simulink model "CompensadorDigitalCorrerArchivoM"  (R2018a)
settings: Solver=VariableStepAuto  StartTime=0.0  StopTime=10.0  RelTol=1e-3
undefined symbols (not defined in the file or in its folder): gcompensado, Gtotalw, integradorDigital
settings Model: Creator=Ignacio  LastModifiedBy=Ignacio

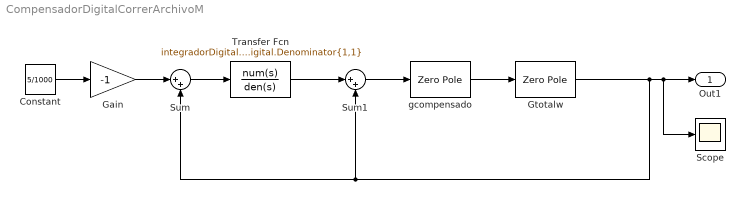
== system CompensadorDigitalCorrerArchivoM ==
  Constant : Constant  Value=5/1000
  Gain : Gain  Gain=-1
  Gtotalw : ZeroPole  Zeros=Gtotalw.Z{1,1}  Poles=Gtotalw.P{1,1}  Gain=Gtotalw.K
  Scope : Scope
  Sum : Sum  Inputs=|++
  Sum1 : Sum  Inputs=|++
  Transfer Fcn : TransferFcn  Numerator=integradorDigital.Numerator{1,1}  Denominator=integradorDigital.Denominator{1,1}
  gcompensado : ZeroPole  Zeros=gcompensado.Z{1,1}  Poles=gcompensado.P{1,1}  Gain=gcompensado.K
  Out1 : Outport
  wires:
  Gtotalw/1 -> Sum1/2, Sum/2, Scope/1, Out1/1
  Transfer Fcn/1 -> Sum1/1
  gcompensado/1 -> Gtotalw/1
  Sum/1 -> Transfer Fcn/1
  Gain/1 -> Sum/1
  Sum1/1 -> gcompensado/1
  Constant/1 -> Gain/1
